simulink model "video2"  (Simulink 7.7)
settings: Solver=ode45  StartTime=0.0  StopTime=10  RelTol=1e-3
undefined symbols (not defined in the file or in its folder): gray, Rec, SDTV
libraries: vipconversions x2, dspsrcs4 x1, vipsnks x1
settings Model: Creator=katsikas  LastModifiedBy=katsikas

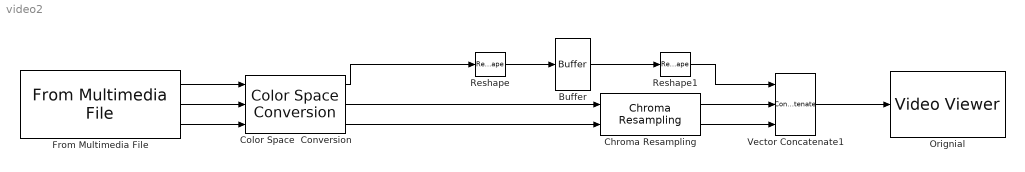
== system video2 ==
  Buffer : Buffer  N=240*160  TreatMby1Signals=One channel
  Chroma Resampling : vipconversions/Chroma Resampling  resampling=4:4:4 to 4:2:2  interpolation=linear  antialiasing=Default  hcoeff=[0.2 0.6 0.2]  vcoeff=[0.5 0.5]  isInputTransposed=off
  Color Space  Conversion : vipconversions/Color Space  Conversion  conversion=Obsolete  conversionActive=R'G'B' to Y'CbCr  wp_str=D65  rec=Rec. 601 (SDTV)  sys=1125/60/2:1  imagePorts=Separate color signals
  From Multimedia File : dspsrcs4/From Multimedia File  inputFilename=/usr/local/MATLAB/R2011a/toolbox/vision/visiondemos/vipunmarkedroad.avi  loop=on  numPlays=inf  outputStreams=Video only  videoDataType=uint8  audioDataType=int16  inheritSampleTime=on  userDefinedSampleTime=1/550  noAudioOutput=off  isIntensityVideo=off  fourcc=RGB  colorVideoFormat=Separate color signals  outputEOF=off  dataOrg=Column-major  audioFrameSize=1024  computeAudioFrameSize=off
  Orignial : vipsnks/Video Viewer  inputType=Obsolete7b  imagePorts=One multidimensional signal  useColorMap=off  colormapValue=gray(256)  specRange=off  minInputVal=0  maxInputVal=255  FigPos=[867 297 170 136]  AxisZoom=on  trueSizedOnce=on  OpenAtMdlStart=on
  Reshape : Reshape  OutputDimensions=[120,160]
  Reshape1 : Reshape  OutputDimensionality=Customize  OutputDimensions=[240,160]
  Vector Concatenate1 : Concatenate  NumInputs=3  Mode=Multidimensional array  ConcatenateDimension=2
  wires:
  From Multimedia File/1 -> Color Space  Conversion/1
  From Multimedia File/2 -> Color Space  Conversion/2
  From Multimedia File/3 -> Color Space  Conversion/3
  Color Space  Conversion/2 -> Chroma Resampling/1
  Color Space  Conversion/3 -> Chroma Resampling/2
  Vector Concatenate1/1 -> Orignial/1
  Color Space  Conversion/1 -> Reshape/1
  Chroma Resampling/2 -> Vector Concatenate1/3
  Chroma Resampling/1 -> Vector Concatenate1/2
  Reshape/1 -> Buffer/1
  Reshape1/1 -> Vector Concatenate1/1
  Buffer/1 -> Reshape1/1
